simulink model "unlinear"  (R2024b)
settings: Solver=VariableStepAuto  StartTime=0.0  StopTime=10  RelTol=1e-3
values from neighbouring files (symbols this model uses):
  Ue = 72.1687836487032*pi    (= 226.724920529)    [prjB1.m]
  X1e = 2*pi/3    (= 2.09439510239)    [prjB1.m]
libraries: cstblocks x1
settings Model: Creator=manucoacci  LastModifiedBy=manucoacci

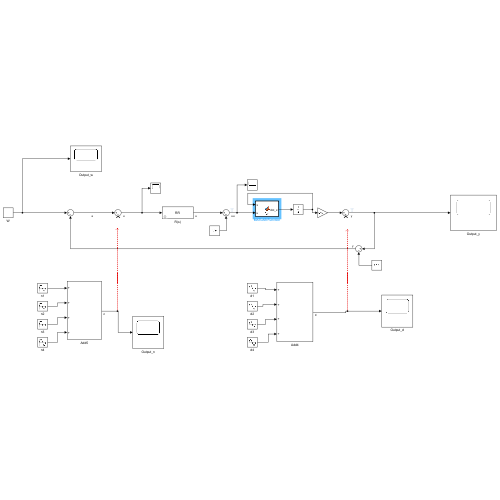
[thumbnail: Simulink's stored preview of the top-level diagram]
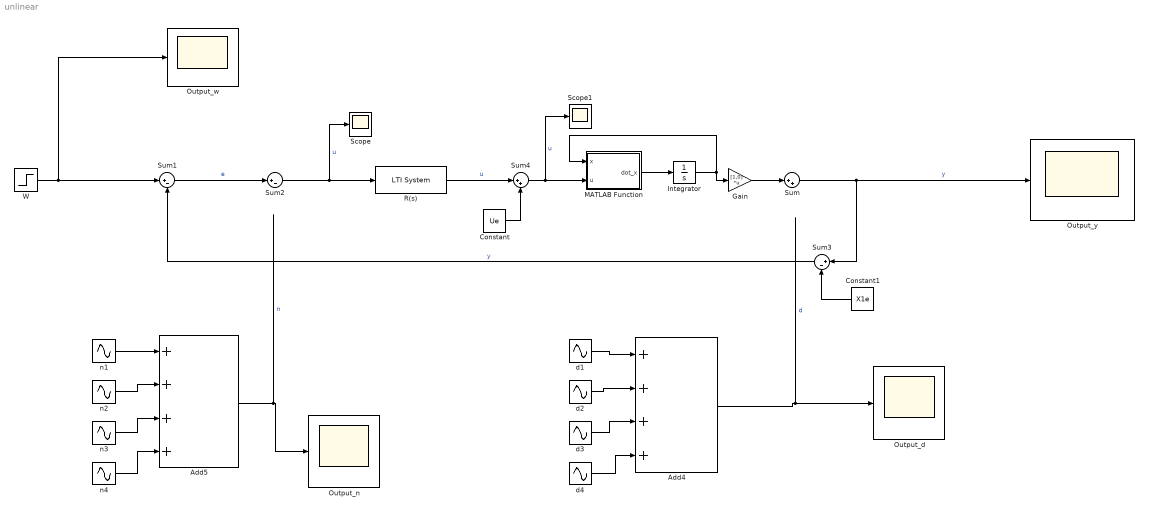
== system unlinear ==
  Add4 : Sum  Inputs=++++
  Add5 : Sum  Inputs=++++
  Constant : Constant  Value=Ue
  Constant1 : Constant  Value=X1e
  Gain : Gain  Gain=[1,0]  Multiplication=Matrix(K*u)
  Integrator : Integrator  InitialCondition=[X1e; 0]
  MATLAB Function : MATLAB Function  TreatAsAtomicUnit=on
  Output_d : Scope
  Output_n : Scope
  Output_w : Scope
  Output_y : Scope
  R(s) : cstblocks/LTI System  sys=RR  IC=[]  PadeOrder=0
  Scope : Scope
  Scope1 : Scope
  Sum : Sum  Inputs=|++
  Sum1 : Sum  Inputs=|+-
  Sum2 : Sum  Inputs=|+-
  Sum3 : Sum  Inputs=|+-
  Sum4 : Sum  Inputs=|++
  W : Step  Time=0  SampleTime=0
  d1 : Sin  Amplitude=0.2  Frequency=0.1*1  SampleTime=0
  d2 : Sin  Amplitude=0.2  Frequency=0.1*2  SampleTime=0
  d3 : Sin  Amplitude=0.2  Frequency=0.1*3  SampleTime=0
  d4 : Sin  Amplitude=0.2  Frequency=0.1*4  SampleTime=0
  n1 : Sin  Amplitude=0.2  Frequency=10000*1  SampleTime=0
  n2 : Sin  Amplitude=0.2  Frequency=10000*2  SampleTime=0
  n3 : Sin  Amplitude=0.2  Frequency=10000*3  SampleTime=0
  n4 : Sin  Amplitude=0.2  Frequency=10000*4  SampleTime=0
  wires:
  d3/1 -> Add4/3
  n4/1 -> Add5/4
  Add5/1 -> Output_n/1  "n"
  n1/1 -> Add5/1
  Sum1/1 -> Sum2/1  "e"
  n3/1 -> Add5/3
  Sum/1 -> Sum3/1, Output_y/1  "y"
  d4/1 -> Add4/4
  d2/1 -> Add4/2
  d1/1 -> Add4/1
  n2/1 -> Add5/2
  W/1 -> Sum1/1, Output_w/1
  Add4/1 -> Output_d/1  "d"
  Gain/1 -> Sum/1
  MATLAB Function/1(dot_x) -> Integrator/1
  Integrator/1 -> MATLAB Function/1(x), Gain/1
  Constant1/1 -> Sum3/2
  Sum3/1 -> Sum1/2  "y"
  Constant/1 -> Sum4/2
  R(s)/1 -> Sum4/1  "u"
  Sum2/1 -> Scope/1, R(s)/1  "u"
  Sum4/1 -> Scope1/1, MATLAB Function/2(u)  "u"

== matlab function unlinear/MATLAB Function ==
  data: x input; u input; dot_x output
function dot_x = fcn(x,u)

%parametri del sistema
k = 100;
beta = 0.6;
alfa = deg2rad(30);
J = 800;


dot_x = zeros(2,1);

dot_x(1) = x(2);
dot_x(2) = (cos(alfa)/(1-(sin(alfa)*cos(x(1)))^2))*u-beta*x(2)-k*x(1);

%dot_x(2) = (cos(alfa)/(1-(sin(alfa)*cos(x(1)))^2)) * u - beta*x(2) - k*x(1) ;
